simulink model "Simulink_Lab1"  (R2022b)
settings: Solver=VariableStepAuto  StartTime=0.0  StopTime=10.0  RelTol=1e-3
settings Model: Creator=dell  LastModifiedBy=dell

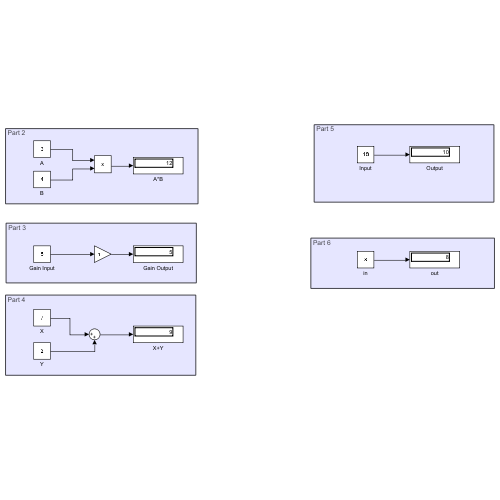
[thumbnail: Simulink's stored preview of the top-level diagram]
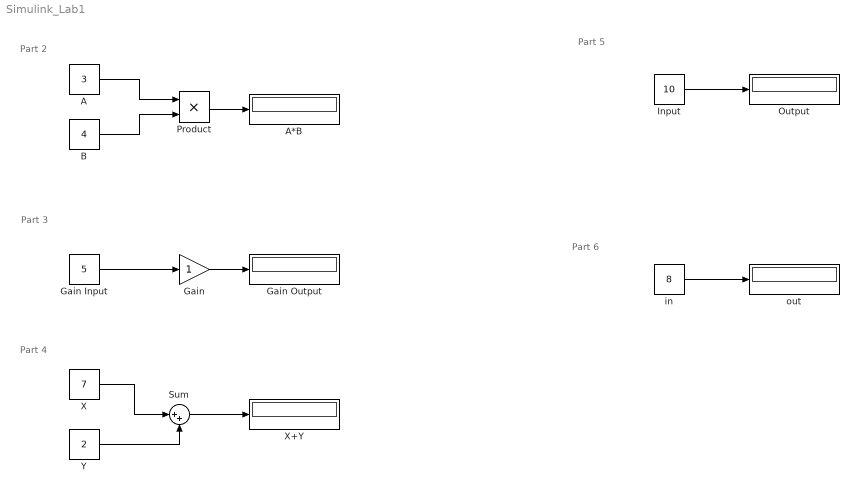
== system Simulink_Lab1 ==
  note: Part 6
  note: Part 5
  note: Part 4
  note: Part 3
  note: Part 2
  A : Constant  Value=3
  A*B : Display
  B : Constant  Value=4
  Gain : Gain
  Gain Input : Constant  Value=5
  Gain Output : Display
  Input : Constant  Value=10
  Output : Display
  Product : Product
  Sum : Sum  Inputs=|++
  X : Constant  Value=7
  X+Y : Display
  Y : Constant  Value=2
  in : Constant  Value=8
  out : Display
  wires:
  Product/1 -> A*B/1
  A/1 -> Product/1
  B/1 -> Product/2
  Gain Input/1 -> Gain/1
  Gain/1 -> Gain Output/1
  X/1 -> Sum/1
  Y/1 -> Sum/2
  Sum/1 -> X+Y/1
  Input/1 -> Output/1
  in/1 -> out/1
